simulink model "model_hil"  (R2016a)
settings: Solver=VariableStepAuto  StartTime=0.0  StopTime=tsim  RelTol=1e-3
values from neighbouring files (symbols this model uses):
  alpha = 0*pi/180    (= 0)    [RunHILsim.m]    (also in RunSimulation.m; plotFrame.m = 0.196349540849; simulation.m)
  b = 0    [Chassis_ss.m]    (also in simulation.m = 0.005)
  c = 0    [Chassis_ss.m]    (also in simulation.m = 0.005)
  CPR = 660    [ControllerDesign.m]
  g = 9.81    [RunHILsim.m]    (also in RunSimulation.m; simulation.m = 9.82)
  I = 0.007358820323616 - M*l^2    (= 0.00237702032362)    [Chassis_ss.m]    (also in simulation.m = 7.8125e-05)
  J = ML_J + MR_J    (= -8.16854715147e-07)    [Chassis_ss.m]    (also in simulation.m = 3.22e-06)
  l = 95e-3    (= 0.095)    [Chassis_ss.m]    (also in simulation.m = 0.5)
  M = 552e-3    (= 0.552)    [Chassis_ss.m]    (also in simulation.m = 1)
  m = 452e-3    (= 0.452)    [Chassis_ss.m]    (also in simulation.m = 0.5)
  ML_Eta = 0.585848927300825    (= 0.585848927301)    [ControllerDesign.m]
  ML_K = 0.009391068653512    (= 0.00939106865351)    [ControllerDesign.m]
  ML_L = 8.62835e-4    (= 0.000862835)    [ControllerDesign.m]
  ML_N = 30    [ControllerDesign.m]
  ML_R = 6.2    [ControllerDesign.m]
  MR_Eta = 0.665816712746634    (= 0.665816712747)    [ControllerDesign.m]
  MR_K = 0.009237618864813    (= 0.00923761886481)    [ControllerDesign.m]
  MR_L = 8.62835e-4    (= 0.000862835)    [ControllerDesign.m]
  MR_N = 30    [ControllerDesign.m]
  MR_R = 6.7    [ControllerDesign.m]
  r = (81.16*10^-3)/2    (= 0.04058)    [Chassis_ss.m]    (also in atan2lookup.m = 1; plotFrame.m = 0.045; simulation.m = 0.045)
  T_kfcorr = 1/200    (= 0.005)    [ControllerDesign.m]
  T_pend = 1/200    (= 0.005)    [ControllerDesign.m]
  theta0 = 25 * pi/180    (= 0.436332312999)    [RunHILsim.m]    (also in RunSimulation.m; simulation.m = 0.0872664625997)
  Vmax = 12    [ControllerDesign.m]
  vref_step_point = 500e-3    (= 0.5)    [RunHILsim.m]    (also in RunSimulation.m)
libraries: instrumentlib x14, simulink x2
settings Model: Creator=masom  LastModifiedBy=masom

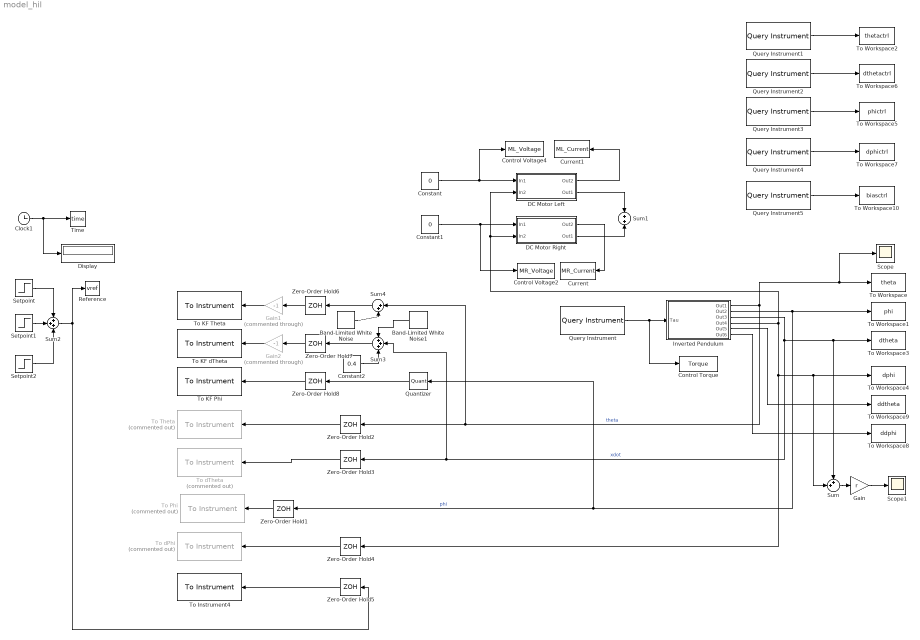
== system model_hil ==
  Band-Limited White Noise : simulink/Sources/Band-Limited White Noise  Cov=[0.000001]  Ts=T_kfcorr  seed=[23341]
  Band-Limited White Noise1 : simulink/Sources/Band-Limited White Noise  Cov=[0.0001]  Ts=T_kfcorr  seed=[10000]
  Clock1 : Clock
  Constant : Constant  Value=0
  Constant1 : Constant  Value=0
  Constant2 : Constant  Value=0.4
  Control Torque : ToWorkspace  VariableName=Torque  SaveFormat=Timeseries  SampleTime=-1
  Control Voltage2 : ToWorkspace  VariableName=MR_Voltage  SaveFormat=Timeseries  SampleTime=-1
  Control Voltage4 : ToWorkspace  VariableName=ML_Voltage  SaveFormat=Timeseries  SampleTime=-1
  Current : ToWorkspace  VariableName=MR_Current  SampleTime=-1
  Current1 : ToWorkspace  VariableName=ML_Current  SampleTime=-1
  DC Motor Left : Subsystem
  DC Motor Right : Subsystem
  Display : Display
  Gain : Gain  Gain=r
  Gain1 : Gain  Commented=through  Gain=-1
  Gain2 : Gain  Commented=through  Gain=-1
  Inverted Pendulum : Subsystem
  Quantizer : Quantizer  QuantizationInterval=1/CPR
  Query Instrument : instrumentlib/Query Instrument  Priority=0  sampleTime=T_pend  isWorkspaceObject=off  timeout=1  inputBufferSize=512  protocol=Serial  serialPort=COM1  baudRate=115200  gpibVendor=Agilent Technologies  boardIndex=0  primaryAddress=1  secondaryAddress=0  visaVendor=Agilent  visaSerialPort=0  chassisIndex=0  logicalAddress=0  tcpRemoteHost='127.0.0.1'  tcpRemotePort=4500  udpRemoteHost='127.0.0.1'  udpRemotePort=9090  visaTCPBoardIndex=0  visaTCPRemoteHost='127.0.0.1'  usbBoardIndex=0  usbManufID=0  usbModelCode=0  usbSerialNumber=0  initAction=None  initCommand='DATA:SOURCE CH1'  initFunction=get  queryCommand='ctrl run KFTIME\nctrl run PEND\n'  responseFormat=ASCII  asciiFormatting='%f\n'  precision=8-bit integer  byteOrder=Little Endian  valuesToRead=1  removeBytes=off  afterOutputAction=Repeat query for new data  enableFrames=off  frameSize=1
  Query Instrument1 : instrumentlib/Query Instrument  Priority=0  sampleTime=T_pend  isWorkspaceObject=off  timeout=10  inputBufferSize=512  protocol=Serial  serialPort=COM1  baudRate=115200  gpibVendor=Agilent Technologies  boardIndex=0  primaryAddress=1  secondaryAddress=0  visaVendor=Agilent  visaSerialPort=0  chassisIndex=0  logicalAddress=0  tcpRemoteHost='127.0.0.1'  tcpRemotePort=4500  udpRemoteHost='127.0.0.1'  udpRemotePort=9090  visaTCPBoardIndex=0  visaTCPRemoteHost='127.0.0.1'  usbBoardIndex=0  usbManufID=0  usbModelCode=0  usbSerialNumber=0  initAction=None  initCommand='DATA:SOURCE CH1'  initFunction=get  queryCommand='ctrl get theta\n'  responseFormat=ASCII  asciiFormatting='theta: %f\n'  precision=8-bit integer  byteOrder=Little Endian  valuesToRead=1  removeBytes=off  afterOutputAction=Repeat query for new data  enableFrames=off  frameSize=1
  Query Instrument2 : instrumentlib/Query Instrument  Priority=0  sampleTime=T_pend  isWorkspaceObject=off  timeout=10  inputBufferSize=512  protocol=Serial  serialPort=COM1  baudRate=115200  gpibVendor=Agilent Technologies  boardIndex=0  primaryAddress=1  secondaryAddress=0  visaVendor=Agilent  visaSerialPort=0  chassisIndex=0  logicalAddress=0  tcpRemoteHost='127.0.0.1'  tcpRemotePort=4500  udpRemoteHost='127.0.0.1'  udpRemotePort=9090  visaTCPBoardIndex=0  visaTCPRemoteHost='127.0.0.1'  usbBoardIndex=0  usbManufID=0  usbModelCode=0  usbSerialNumber=0  initAction=None  initCommand='DATA:SOURCE CH1'  initFunction=get  queryCommand='ctrl get dtheta\n'  responseFormat=ASCII  asciiFormatting='dtheta: %f\n'  precision=8-bit integer  byteOrder=Little Endian  valuesToRead=1  removeBytes=off  afterOutputAction=Repeat query for new data  enableFrames=off  frameSize=1
  Query Instrument3 : instrumentlib/Query Instrument  Priority=0  sampleTime=T_pend  isWorkspaceObject=off  timeout=10  inputBufferSize=512  protocol=Serial  serialPort=COM1  baudRate=115200  gpibVendor=Agilent Technologies  boardIndex=0  primaryAddress=1  secondaryAddress=0  visaVendor=Agilent  visaSerialPort=0  chassisIndex=0  logicalAddress=0  tcpRemoteHost='127.0.0.1'  tcpRemotePort=4500  udpRemoteHost='127.0.0.1'  udpRemotePort=9090  visaTCPBoardIndex=0  visaTCPRemoteHost='127.0.0.1'  usbBoardIndex=0  usbManufID=0  usbModelCode=0  usbSerialNumber=0  initAction=None  initCommand='DATA:SOURCE CH1'  initFunction=get  queryCommand='ctrl get phi\n'  responseFormat=ASCII  asciiFormatting='phi: %f\n'  precision=8-bit integer  byteOrder=Little Endian  valuesToRead=1  removeBytes=off  afterOutputAction=Repeat query for new data  enableFrames=off  frameSize=1
  Query Instrument4 : instrumentlib/Query Instrument  Priority=0  sampleTime=T_pend  isWorkspaceObject=off  timeout=10  inputBufferSize=512  protocol=Serial  serialPort=COM1  baudRate=115200  gpibVendor=Agilent Technologies  boardIndex=0  primaryAddress=1  secondaryAddress=0  visaVendor=Agilent  visaSerialPort=0  chassisIndex=0  logicalAddress=0  tcpRemoteHost='127.0.0.1'  tcpRemotePort=4500  udpRemoteHost='127.0.0.1'  udpRemotePort=9090  visaTCPBoardIndex=0  visaTCPRemoteHost='127.0.0.1'  usbBoardIndex=0  usbManufID=0  usbModelCode=0  usbSerialNumber=0  initAction=None  initCommand='DATA:SOURCE CH1'  initFunction=get  queryCommand='ctrl get dphi\n'  responseFormat=ASCII  asciiFormatting='dphi: %f\n'  precision=8-bit integer  byteOrder=Little Endian  valuesToRead=1  removeBytes=off  afterOutputAction=Repeat query for new data  enableFrames=off  frameSize=1
  Query Instrument5 : instrumentlib/Query Instrument  Priority=0  sampleTime=T_pend  isWorkspaceObject=off  timeout=10  inputBufferSize=512  protocol=Serial  serialPort=COM1  baudRate=115200  gpibVendor=Agilent Technologies  boardIndex=0  primaryAddress=1  secondaryAddress=0  visaVendor=Agilent  visaSerialPort=0  chassisIndex=0  logicalAddress=0  tcpRemoteHost='127.0.0.1'  tcpRemotePort=4500  udpRemoteHost='127.0.0.1'  udpRemotePort=9090  visaTCPBoardIndex=0  visaTCPRemoteHost='127.0.0.1'  usbBoardIndex=0  usbManufID=0  usbModelCode=0  usbSerialNumber=0  initAction=None  initCommand='DATA:SOURCE CH1'  initFunction=get  queryCommand='ctrl get bias\n'  responseFormat=ASCII  asciiFormatting='bias: %f\n'  precision=8-bit integer  byteOrder=Little Endian  valuesToRead=1  removeBytes=off  afterOutputAction=Repeat query for new data  enableFrames=off  frameSize=1
  Reference : ToWorkspace  VariableName=vref  SaveFormat=Timeseries  SampleTime=-1
  Scope : Scope
  Scope1 : Scope
  Setpoint : Step  Time=10  After=vref_step_point  SampleTime=0
  Setpoint1 : Step  Time=11.5  After=-2*vref_step_point  SampleTime=0
  Setpoint2 : Step  Time=20  After=vref_step_point  SampleTime=0
  Sum : Sum  Inputs=++|
  Sum1 : Sum  Inputs=+|+
  Sum2 : Sum  Inputs=+++
  Sum3 : Sum  Inputs=+++
  Sum4 : Sum  Inputs=|++
  Time : ToWorkspace  VariableName=time  SampleTime=-1
  To Instrument4 : instrumentlib/To Instrument  Priority=3  sampleTime=-1  isWorkspaceObject=off  timeout=10  inputBufferSize=8192  protocol=Serial  serialPort=COM1  baudRate=115200  gpibVendor=Agilent Technologies  boardIndex=0  primaryAddress=1  secondaryAddress=0  visaVendor=Agilent  visaSerialPort=0  chassisIndex=0  logicalAddress=0  tcpRemoteHost='127.0.0.1'  tcpRemotePort=4500  udpRemoteHost='127.0.0.1'  udpRemotePort=9090  visaTCPBoardIndex=0  visaTCPRemoteHost='127.0.0.1'  usbBoardIndex=0  usbManufID=0  usbModelCode=0  usbSerialNumber=0  initAction=None  initCommand='DATA:SOURCE CH1'  initFunction=get  command=''  sendFormat=ASCII  asciiFormatting='ctrl set vref %f\n'  precision=8-bit integer  byteOrder=Little Endian
  To KF Phi : instrumentlib/To Instrument  Priority=2  sampleTime=-1  isWorkspaceObject=off  timeout=10  inputBufferSize=8192  protocol=Serial  serialPort=COM1  baudRate=115200  gpibVendor=Agilent Technologies  boardIndex=0  primaryAddress=1  secondaryAddress=0  visaVendor=Agilent  visaSerialPort=0  chassisIndex=0  logicalAddress=0  tcpRemoteHost='127.0.0.1'  tcpRemotePort=4500  udpRemoteHost='127.0.0.1'  udpRemotePort=9090  visaTCPBoardIndex=0  visaTCPRemoteHost='127.0.0.1'  usbBoardIndex=0  usbManufID=0  usbModelCode=0  usbSerialNumber=0  initAction=None  initCommand='DATA:SOURCE CH1'  initFunction=get  command=''  sendFormat=ASCII  asciiFormatting='ctrl correct phi %f\n'  precision=8-bit integer  byteOrder=Little Endian
  To KF Theta : instrumentlib/To Instrument  Priority=4  sampleTime=-1  isWorkspaceObject=off  timeout=10  inputBufferSize=8192  protocol=Serial  serialPort=COM1  baudRate=115200  gpibVendor=Agilent Technologies  boardIndex=0  primaryAddress=1  secondaryAddress=0  visaVendor=Agilent  visaSerialPort=0  chassisIndex=0  logicalAddress=0  tcpRemoteHost='127.0.0.1'  tcpRemotePort=4500  udpRemoteHost='127.0.0.1'  udpRemotePort=9090  visaTCPBoardIndex=0  visaTCPRemoteHost='127.0.0.1'  usbBoardIndex=0  usbManufID=0  usbModelCode=0  usbSerialNumber=0  initAction=None  initCommand='ctrl mode HIL\n'  initFunction=get  command=''  sendFormat=ASCII  asciiFormatting='ctrl correct theta %f\n'  precision=8-bit integer  byteOrder=Little Endian
  To KF dTheta : instrumentlib/To Instrument  Priority=1  sampleTime=-1  isWorkspaceObject=off  timeout=10  inputBufferSize=8192  protocol=Serial  serialPort=COM1  baudRate=115200  gpibVendor=Agilent Technologies  boardIndex=0  primaryAddress=1  secondaryAddress=0  visaVendor=Agilent  visaSerialPort=0  chassisIndex=0  logicalAddress=0  tcpRemoteHost='127.0.0.1'  tcpRemotePort=4500  udpRemoteHost='127.0.0.1'  udpRemotePort=9090  visaTCPBoardIndex=0  visaTCPRemoteHost='127.0.0.1'  usbBoardIndex=0  usbManufID=0  usbModelCode=0  usbSerialNumber=0  initAction=None  initCommand='DATA:SOURCE CH1'  initFunction=get  command=''  sendFormat=ASCII  asciiFormatting='ctrl correct dtheta %f\n'  precision=8-bit integer  byteOrder=Little Endian
  To Phi : instrumentlib/To Instrument  Commented=on  sampleTime=-1  isWorkspaceObject=off  timeout=10  inputBufferSize=8192  protocol=Serial  serialPort=COM1  baudRate=115200  gpibVendor=Agilent Technologies  boardIndex=0  primaryAddress=1  secondaryAddress=0  visaVendor=Agilent  visaSerialPort=0  chassisIndex=0  logicalAddress=0  tcpRemoteHost='127.0.0.1'  tcpRemotePort=4500  udpRemoteHost='127.0.0.1'  udpRemotePort=9090  visaTCPBoardIndex=0  visaTCPRemoteHost='127.0.0.1'  usbBoardIndex=0  usbManufID=0  usbModelCode=0  usbSerialNumber=0  initAction=None  initCommand='DATA:SOURCE CH1'  initFunction=get  command=''  sendFormat=ASCII  asciiFormatting='ctrl set phi %d\n'  precision=8-bit integer  byteOrder=Little Endian
  To Theta : instrumentlib/To Instrument  Priority=4  Commented=on  sampleTime=-1  isWorkspaceObject=off  timeout=10  inputBufferSize=8192  protocol=Serial  serialPort=COM1  baudRate=115200  gpibVendor=Agilent Technologies  boardIndex=0  primaryAddress=1  secondaryAddress=0  visaVendor=Agilent  visaSerialPort=0  chassisIndex=0  logicalAddress=0  tcpRemoteHost='127.0.0.1'  tcpRemotePort=4500  udpRemoteHost='127.0.0.1'  udpRemotePort=9090  visaTCPBoardIndex=0  visaTCPRemoteHost='127.0.0.1'  usbBoardIndex=0  usbManufID=0  usbModelCode=0  usbSerialNumber=0  initAction=None  initCommand='ctrl mode HIL\n'  initFunction=get  command=''  sendFormat=ASCII  asciiFormatting='ctrl set theta %f\n'  precision=8-bit integer  byteOrder=Little Endian
  To Workspace : ToWorkspace  VariableName=theta  SaveFormat=Timeseries  SampleTime=-1
  To Workspace1 : ToWorkspace  VariableName=phi  SaveFormat=Timeseries  SampleTime=-1
  To Workspace10 : ToWorkspace  VariableName=biasctrl  SaveFormat=Timeseries  SampleTime=-1
  To Workspace2 : ToWorkspace  VariableName=thetactrl  SaveFormat=Timeseries  SampleTime=-1
  To Workspace3 : ToWorkspace  VariableName=dtheta  SaveFormat=Timeseries  SampleTime=-1
  To Workspace4 : ToWorkspace  VariableName=dphi  SaveFormat=Timeseries  SampleTime=-1
  To Workspace5 : ToWorkspace  VariableName=phictrl  SaveFormat=Timeseries  SampleTime=-1
  To Workspace6 : ToWorkspace  VariableName=dthetactrl  SaveFormat=Timeseries  SampleTime=-1
  To Workspace7 : ToWorkspace  VariableName=dphictrl  SaveFormat=Timeseries  SampleTime=-1
  To Workspace8 : ToWorkspace  VariableName=ddphi  SaveFormat=Timeseries  SampleTime=-1
  To Workspace9 : ToWorkspace  VariableName=ddtheta  SaveFormat=Timeseries  SampleTime=-1
  To dPhi : instrumentlib/To Instrument  Priority=2  Commented=on  sampleTime=-1  isWorkspaceObject=off  timeout=10  inputBufferSize=8192  protocol=Serial  serialPort=COM1  baudRate=115200  gpibVendor=Agilent Technologies  boardIndex=0  primaryAddress=1  secondaryAddress=0  visaVendor=Agilent  visaSerialPort=0  chassisIndex=0  logicalAddress=0  tcpRemoteHost='127.0.0.1'  tcpRemotePort=4500  udpRemoteHost='127.0.0.1'  udpRemotePort=9090  visaTCPBoardIndex=0  visaTCPRemoteHost='127.0.0.1'  usbBoardIndex=0  usbManufID=0  usbModelCode=0  usbSerialNumber=0  initAction=None  initCommand='DATA:SOURCE CH1'  initFunction=get  command=''  sendFormat=ASCII  asciiFormatting='ctrl set dphi %f\n'  precision=8-bit integer  byteOrder=Little Endian
  To dTheta : instrumentlib/To Instrument  Priority=1  Commented=on  sampleTime=-1  isWorkspaceObject=off  timeout=10  inputBufferSize=8192  protocol=Serial  serialPort=COM1  baudRate=115200  gpibVendor=Agilent Technologies  boardIndex=0  primaryAddress=1  secondaryAddress=0  visaVendor=Agilent  visaSerialPort=0  chassisIndex=0  logicalAddress=0  tcpRemoteHost='127.0.0.1'  tcpRemotePort=4500  udpRemoteHost='127.0.0.1'  udpRemotePort=9090  visaTCPBoardIndex=0  visaTCPRemoteHost='127.0.0.1'  usbBoardIndex=0  usbManufID=0  usbModelCode=0  usbSerialNumber=0  initAction=None  initCommand='DATA:SOURCE CH1'  initFunction=get  command=''  sendFormat=ASCII  asciiFormatting='ctrl set dtheta %f\n'  precision=8-bit integer  byteOrder=Little Endian
  Zero-Order Hold{1..5} (5 alike) : ZeroOrderHold  SampleTime=T_pend
  Zero-Order Hold6 : ZeroOrderHold  SampleTime=T_kfcorr
  Zero-Order Hold7 : ZeroOrderHold  SampleTime=T_kfcorr
  Zero-Order Hold8 : ZeroOrderHold  SampleTime=T_kfcorr
  wires:
  Inverted Pendulum/2(Out2) -> Zero-Order Hold1/1, Quantizer/1, To Workspace1/1  "phi"
  Clock1/1 -> Display/1, Time/1
  Inverted Pendulum/1(Out1) -> Sum4/1, Zero-Order Hold2/1, Scope/1, To Workspace/1  "theta"
  Setpoint/1 -> Sum2/1
  Setpoint1/1 -> Sum2/2
  Sum2/1 -> Zero-Order Hold5/1, Reference/1
  Inverted Pendulum/3(Out3) -> Sum/1, To Workspace3/1, Sum3/2, Zero-Order Hold3/1  "xdot"
  Inverted Pendulum/5(Out5) -> To Workspace9/1
  Inverted Pendulum/6(Out6) -> To Workspace8/1
  Inverted Pendulum/4(Out4) -> Sum/2, To Workspace4/1, Zero-Order Hold4/1, DC Motor Left/2(In2), DC Motor Right/2(In2)
  DC Motor Right/2(Out1) -> Sum1/2
  Setpoint2/1 -> Sum2/3
  DC Motor Left/2(Out1) -> Sum1/1
  Zero-Order Hold3/1 -> To dTheta/1
  Zero-Order Hold4/1 -> To dPhi/1
  Zero-Order Hold5/1 -> To Instrument4/1
  Query Instrument/1 -> Control Torque/1, Inverted Pendulum/1(Tau)
  Zero-Order Hold2/1 -> To Theta/1
  Zero-Order Hold1/1 -> To Phi/1
  Sum/1 -> Gain/1
  Gain/1 -> Scope1/1
  DC Motor Left/1(Out2) -> Current1/1
  Constant/1 -> Control Voltage4/1, DC Motor Left/1(In1)
  Constant1/1 -> Control Voltage2/1, DC Motor Right/1(In1)
  DC Motor Right/1(Out2) -> Current/1
  Query Instrument4/1 -> To Workspace7/1
  Query Instrument2/1 -> To Workspace6/1
  Query Instrument1/1 -> To Workspace2/1
  Query Instrument3/1 -> To Workspace5/1
  Zero-Order Hold7/1 -> Gain2/1
  Zero-Order Hold8/1 -> To KF Phi/1
  Zero-Order Hold6/1 -> Gain1/1
  Gain1/1 -> To KF Theta/1
  Gain2/1 -> To KF dTheta/1
  Sum3/1 -> Zero-Order Hold7/1
  Constant2/1 -> Sum3/3
  Query Instrument5/1 -> To Workspace10/1
  Sum4/1 -> Zero-Order Hold6/1
  Band-Limited White Noise1/1 -> Sum3/1
  Band-Limited White Noise/1 -> Sum4/2
  Quantizer/1 -> Zero-Order Hold8/1

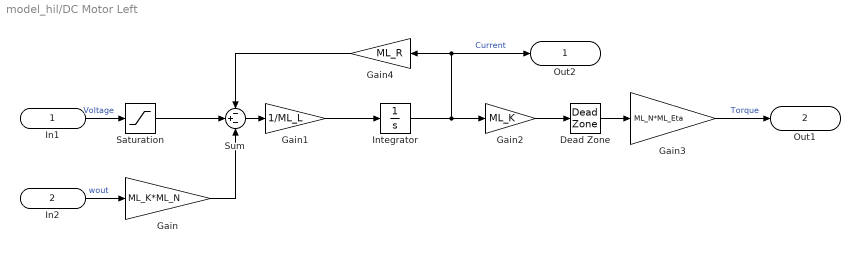
== system model_hil/DC Motor Left ==
  In1 : Inport
  In2 : Inport  Port=2
  Dead Zone : DeadZone  LowerValue=MR_Tm_neg  UpperValue=MR_Tm_pos  SaturateOnIntegerOverflow=on
  Gain : Gain  Gain=ML_K*ML_N
  Gain1 : Gain  Gain=1/ML_L
  Gain2 : Gain  Gain=ML_K
  Gain3 : Gain  Gain=ML_N*ML_Eta
  Gain4 : Gain  Gain=ML_R
  Integrator : Integrator
  Saturation : Saturate  UpperLimit=Vmax  LowerLimit=-Vmax
  Sum : Sum  Inputs=-+-
  Out2 : Outport
  Out1 : Outport  Port=2
  wires:
  Saturation/1 -> Sum/2
  Gain4/1 -> Sum/1
  Integrator/1 -> Gain2/1, Out2/1, Gain4/1  "Current"
  Gain3/1 -> Out1/1  "Torque"
  Dead Zone/1 -> Gain3/1
  Gain2/1 -> Dead Zone/1
  Gain1/1 -> Integrator/1
  Sum/1 -> Gain1/1
  Gain/1 -> Sum/3
  In2/1 -> Gain/1  "wout"
  In1/1 -> Saturation/1  "Voltage"

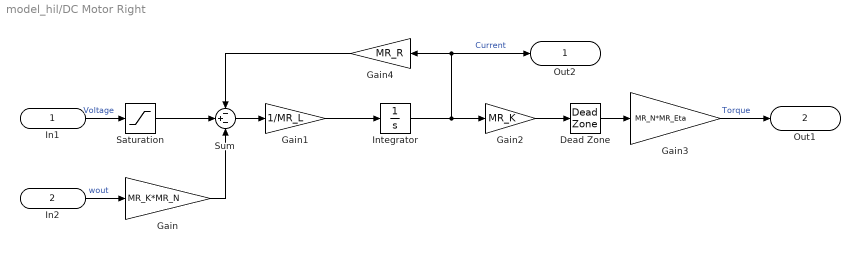
== system model_hil/DC Motor Right ==
  In1 : Inport
  In2 : Inport  Port=2
  Dead Zone : DeadZone  LowerValue=MR_Tm_neg  UpperValue=MR_Tm_pos  SaturateOnIntegerOverflow=on
  Gain : Gain  Gain=MR_K*MR_N
  Gain1 : Gain  Gain=1/MR_L
  Gain2 : Gain  Gain=MR_K
  Gain3 : Gain  Gain=MR_N*MR_Eta
  Gain4 : Gain  Gain=MR_R
  Integrator : Integrator
  Saturation : Saturate  UpperLimit=Vmax  LowerLimit=-Vmax
  Sum : Sum  Inputs=-+-
  Out2 : Outport
  Out1 : Outport  Port=2
  wires:
  In1/1 -> Saturation/1  "Voltage"
  In2/1 -> Gain/1  "wout"
  Gain/1 -> Sum/3
  Sum/1 -> Gain1/1
  Gain1/1 -> Integrator/1
  Gain2/1 -> Dead Zone/1
  Dead Zone/1 -> Gain3/1
  Gain3/1 -> Out1/1  "Torque"
  Integrator/1 -> Gain4/1, Out2/1, Gain2/1  "Current"
  Gain4/1 -> Sum/1
  Saturation/1 -> Sum/2

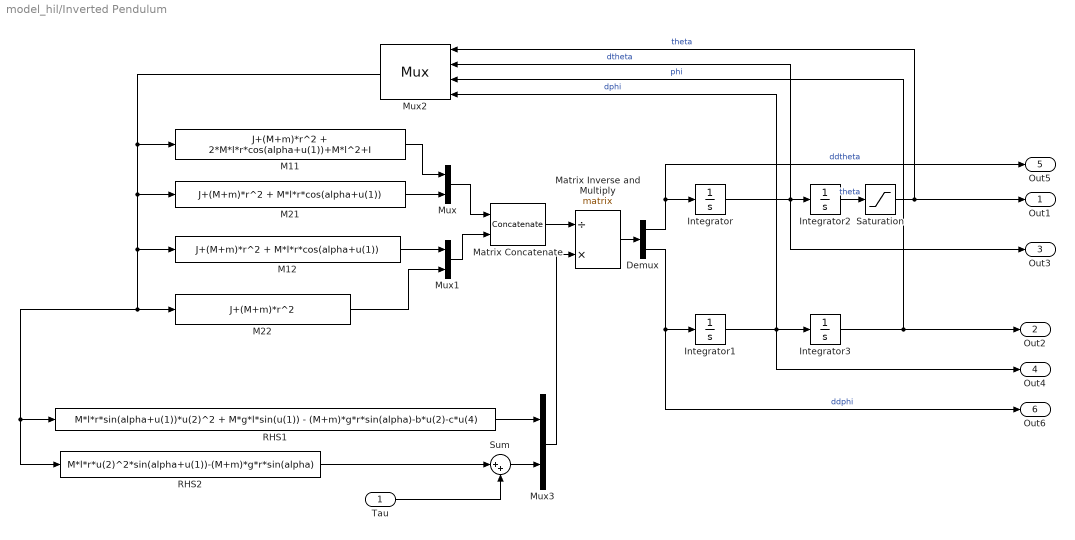
== system model_hil/Inverted Pendulum ==
  Tau : Inport
  Demux : Demux  Outputs=2
  Integrator : Integrator  ContinuousStateAttributes='dtheta'
  Integrator1 : Integrator  ContinuousStateAttributes='dphi'
  Integrator2 : Integrator  InitialCondition=theta0  ContinuousStateAttributes='theta'
  Integrator3 : Integrator  ContinuousStateAttributes='phi'
  M11 : Fcn  Expr=J+(M+m)*r^2 + 2*M*l*r*cos(alpha+u(1))+M*l^2+I
  M12 : Fcn  Expr=J+(M+m)*r^2 + M*l*r*cos(alpha+u(1))
  "M21 " : Fcn  Expr=J+(M+m)*r^2 + M*l*r*cos(alpha+u(1))
  M22 : Fcn  Expr=J+(M+m)*r^2
  Matrix Concatenate : Concatenate  Mode=Multidimensional array  ConcatenateDimension=2
  Matrix Inverse and Multiply : Product  Inputs=/*  Multiplication=Matrix(*)
  Mux : Mux  Inputs=2
  Mux1 : Mux  Inputs=2
  Mux2 : Mux
      settings: DisplayOption=signals
  Mux3 : Mux  Inputs=2
  RHS1 : Fcn  Expr=M*l*r*sin(alpha+u(1))*u(2)^2 + M*g*l*sin(u(1)) - (M+m)*g*r*sin(alpha)-b*u(2)-c*u(4)
  RHS2 : Fcn  Expr=M*l*r*u(2)^2*sin(alpha+u(1))-(M+m)*g*r*sin(alpha)
  Saturation : Saturate  UpperLimit=pi  LowerLimit=-pi
  Sum : Sum  Inputs=|++
  Out1 : Outport
  Out2 : Outport  Port=2
  Out3 : Outport  Port=3
  Out4 : Outport  Port=4
  Out5 : Outport  Port=5
  Out6 : Outport  Port=6
  wires:
  M12/1 -> Mux1/1
  Integrator1/1 -> Out4/1, Mux2/4, Integrator3/1  "dphi"
  Demux/1 -> Out5/1, Integrator/1  "ddtheta"
  Mux/1 -> Matrix Concatenate/1
  Matrix Concatenate/1 -> Matrix Inverse and Multiply/1
  Demux/2 -> Integrator1/1, Out6/1  "ddphi"
  Mux1/1 -> Matrix Concatenate/2
  RHS2/1 -> Sum/1
  Matrix Inverse and Multiply/1 -> Demux/1
  Sum/1 -> Mux3/2
  Integrator/1 -> Out3/1, Mux2/2, Integrator2/1  "dtheta"
  Integrator2/1 -> Saturation/1  "theta"
  Mux2/1 -> "M21 "/1, M22/1, RHS2/1, RHS1/1, M12/1, M11/1
  Mux3/1 -> Matrix Inverse and Multiply/2
  M11/1 -> Mux/1
  "M21 "/1 -> Mux/2
  Integrator3/1 -> Out2/1, Mux2/3  "phi"
  RHS1/1 -> Mux3/1
  Tau/1 -> Sum/2
  M22/1 -> Mux1/2
  Saturation/1 -> Out1/1, Mux2/1  "theta"
